simulink model "basic_motor"  (R2025a)
settings: Solver=VariableStepAuto  StartTime=0.0  StopTime=1.5  MaxStep=1e-5  RelTol=1e-3
values from neighbouring files (symbols this model uses):
  B = 1.0    (= 1)    [defines_script.m]
  I_step = 5.5    [defines_script.m]
  J = 0.3    [defines_script.m]
  K = 4.0    (= 4)    [defines_script.m]
  K_est = K    (= 4)    [defines_script.m]
  K_ia = 220    [defines_script.m]
  K_pa = 7    [defines_script.m]
  L = 0.011    [defines_script.m]
  R = 0.115    [defines_script.m]
  Tl = 0    [defines_script.m]
settings Model: Creator=lpurd  LastModifiedBy=lpurd

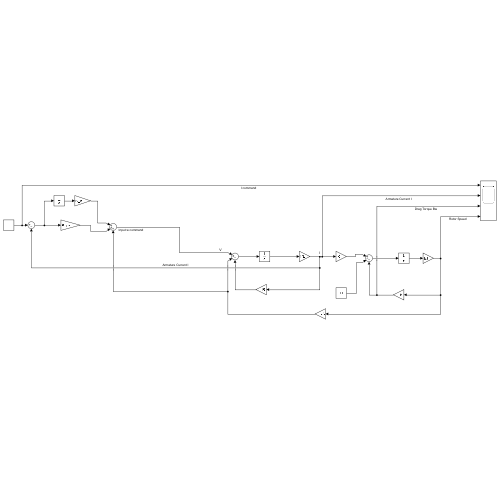
[thumbnail: Simulink's stored preview of the top-level diagram]
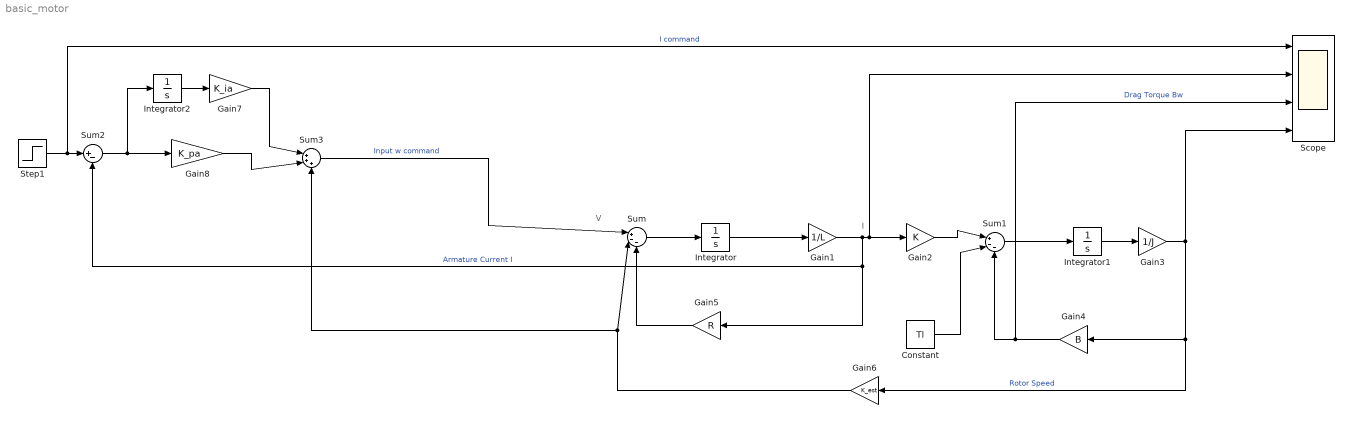
== system basic_motor ==
  note: V
  note: I
  Constant : Constant  Value=Tl
  Gain1 : Gain  Gain=1/L
  Gain2 : Gain  Gain=K
  Gain3 : Gain  Gain=1/J
  Gain4 : Gain  Gain=B
  Gain5 : Gain  Gain=R
  Gain6 : Gain  Gain=K_est
  Gain7 : Gain  Gain=K_ia
  Gain8 : Gain  Gain=K_pa
  Integrator : Integrator
  Integrator1 : Integrator
  Integrator2 : Integrator
  Scope : Scope  NumInputPorts=4
      settings: ActiveDisplayYMinimum=4.5  ActiveDisplayYMaximum=6.5
  Step1 : Step  Time=0  After=I_step  SampleTime=0
  Sum : Sum  Inputs=|+--
  Sum1 : Sum  Inputs=|+--
  Sum2 : Sum  Inputs=|+-
  Sum3 : Sum  Inputs=|+++
  wires:
  Sum/1 -> Integrator/1
  Integrator/1 -> Gain1/1
  Gain1/1 -> Sum2/2, Gain5/1, Scope/2, Gain2/1  "Armature Current I"
  Gain2/1 -> Sum1/1
  Sum1/1 -> Integrator1/1
  Integrator1/1 -> Gain3/1
  Gain3/1 -> Gain6/1, Gain4/1, Scope/4  "Rotor Speed"
  Gain4/1 -> Scope/3, Sum1/3  "Drag Torque Bw"
  Gain5/1 -> Sum/3
  Gain6/1 -> Sum3/3, Sum/2
  Sum3/1 -> Sum/1  "Input w command"
  Constant/1 -> Sum1/2
  Gain7/1 -> Sum3/1
  Gain8/1 -> Sum3/2
  Integrator2/1 -> Gain7/1
  Sum2/1 -> Gain8/1, Integrator2/1
  Step1/1 -> Scope/1, Sum2/1  "I command"
